simulink model "rtwdemo_codetemplate"  (Simulink 7.6)
settings: Solver=FixedStepDiscrete  StartTime=0.0  StopTime=48  FixedStep=1  RelTol=1e-3
libraries: rtwdemowidgets x2, simulink x1
Description:
  | Formatting Generated Files with Templates
settings Model: Creator=The MathWorks Inc.  ModifiedHistory=This text maps to the Code Template %<ModifiedComment> symbol.  ParamWorkspaceSource=ReferencedWorkspace  CovMetricSettings=d  ExtModeTrigMode=oneshot  ExtModeArmWhenConnect=off  ExtModeAutoUpdateStatusClock=off
settings MATStruct: SampleTime=1  Offset=0  Priority=[20.0]
settings DataIOCC: LimitDataPoints=off  SaveFormat=StructureWithTime  SaveOutput=off  SaveTime=off  SignalLoggingName=sigsOut
settings OptimizationCC: InlineParams=on  InlineInvariantSignals=on  PassReuseOutputArgsAs=Individual arguments  StateBitsets=on  DataBitsets=on  UseTempVars=on  ZeroExternalMemoryAtStartup=off  ZeroInternalMemoryAtStartup=off  NoFixptDivByZeroProtection=on  EfficientFloat2IntCast=on  EfficientMapNaN2IntZero=off  OptimizeModelRefInitCode=on  LifeSpan=1  BufferReusableBoundary=off
settings DebuggingCC: CheckExecutionContextPreStartOutputMsg=on  CheckExecutionContextRuntimeOutputMsg=on  SolverPrmCheckMsg=none  IntegerOverflowMsg=none  StrictBusMsg=ErrorOnBusTreatedAsVector
settings HardwareCC: ProdIntDivRoundTo=Zero  ProdEndianess=LittleEndian  ProdHWDeviceType=Generic->32-bit Embedded Processor  TargetHWDeviceType=Generic->32-bit Embedded Processor
settings ModelReferenceCC: UpdateModelReferenceTargets=IfOutOfDate
settings RTWCC: SystemTargetFile=ert.tlc  TLCOptions=-p0 -aWarnNonSaturatedBlocks=0  TemplateMakefile=ert_default_tmf  Description=Real-Time Workshop Embedded Coder (no auto configuration)  GenerateReport=on  RTWVerbose=off  ProcessScript=ert_make_rtw_hook  IncludeHyperlinkInReport=on  LaunchReport=on
settings CodeAppCC: ForceParamTrailComments=on  IgnoreCustomStorageClasses=off  IgnoreTestpoints=on  SimulinkDataObjDesc=on  CustomSymbolStrGlobalVar=rt$N$M  CustomSymbolStrType=$N$M  CustomSymbolStrFcn=$N$M$F  CustomSymbolStrMacro=$N$M  InsertBlockDesc=on
settings ERTTargetCC: TargetFcnLib=ansi_tfl_tmw.mat  MultiwordLength=2048  GenerateSampleERTMain=on  IncludeMdlTerminateFcn=off  SupportNonFinite=off  SupportComplex=off  InlinedParameterPlacement=NonHierarchical  ERTSrcFileBannerTemplate=rtwdemocodetemplate.cgt  ERTHdrFileBannerTemplate=rtwdemocodetemplate.cgt  ERTDataSrcFileTemplate=rtwdemocodetemplate.cgt  ERTDataHdrFileTemplate=rtwdemocodetemplate.cgt  ERTCustomFileTemplate=example_file_process.tlc  ConvertIfToSwitch=off

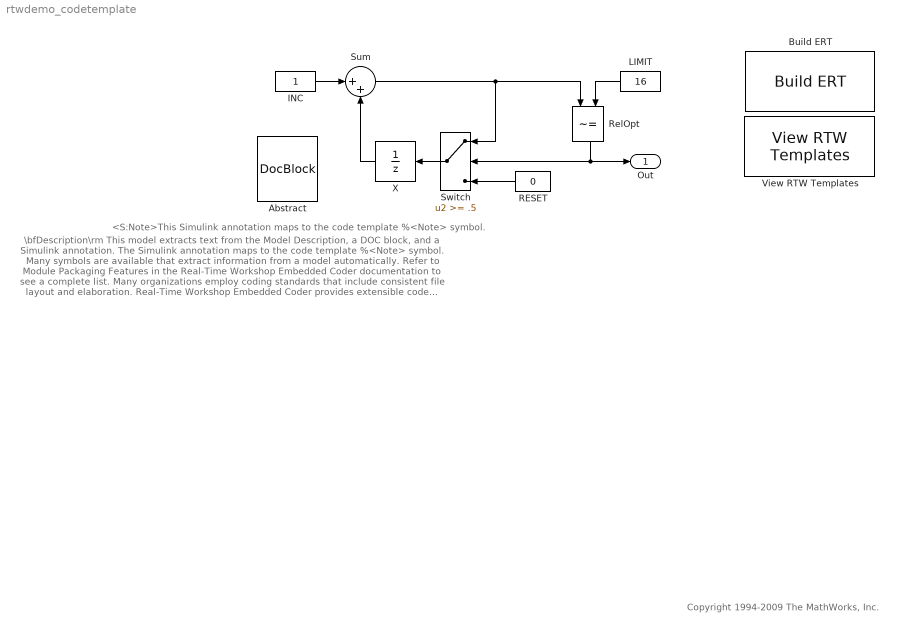
== system rtwdemo_codetemplate ==
  note: \bfDescription\rm
      | This model extracts text from the Model Description, a DOC block, and a Simulink annotation.  The Simulink
      | annotation maps to the code template %<Note> symbol.  Many symbols are available that extract information
      | from a model automatically.  Refer to Module Packaging Features in the Real-Time Workshop Embedded
      | Coder documentation to see a complete list.
      |
      | Many organizations employ coding standards that include consistent file layout and elaboration.  Real-Time
      | Workshop Embedded Coder provides extensible code generation templates for formatting generated code.
      | The layout and format of the code template file controls the output of the generated code.
      |
      | Code generation templates (.cgt files) allow you to add custom code banners, rearrange data and functions,
      | and insert additional code segments and documentation into generated code files.  Code generation
      | templates are picked up automatically from the MATLAB path and employed during the code generation
      | process.  For this model, the code generation template "rtwdemocodetemplate.cgt" is used.
      |
      | \bfInstructions\rm
      | 1. Double-click the yellow View Templates Configuration button to view the templates configuration.
      | 2. Click the Edit button to the right of the "rtwdemocodetemplate.cgt" template, and inspect the code template.
      | 3. Double-click the blue button in the upper right to generate code.  An HTML report appears automatically.
      | 4. Open rtwdemo\_codetemplate.c to inspect the generated code for this model.
  note: <S:Note>This Simulink annotation maps to the code template %<Note> symbol.
  note: Copyright 1994-2009 The MathWorks, Inc.
  Abstract : simulink/Model-Wide Utilities/DocBlock  SystemSampleTime=-1  ECoderFlag=Abstract  DocumentType=Text
      settings: AttributesFormatString=%<ECoderFlag>
  Build ERT : rtwdemowidgets/Build ERT  SystemSampleTime=-1  attrib_overrides={'ERTSrcFileBannerTemplate', 'ERTHdrFileBannerTemplate', 'ERTDataSrcFileTemplate', 'ERTDataHdrFileTemplate'}
  INC : Constant  OutDataTypeStr=uint8
  LIMIT : Constant  Value=16  OutDataTypeStr=uint8
  RESET : Constant  Value=0  OutDataTypeStr=uint8
  RelOpt : RelationalOperator  Operator=~=  InputSameDT=on
  Sum : Sum  Inputs=|++  InputSameDT=on  OutDataTypeStr=Inherit: Same as first input
  Switch : Switch  Threshold=.5  SaturateOnIntegerOverflow=on  InputSameDT=on
  View RTW Templates : rtwdemowidgets/View RTW Templates  SystemSampleTime=-1
  X : UnitDelay  StateIdentifier=X
  Out : Outport
  wires:
  INC/1 -> Sum/1
  X/1 -> Sum/2
  Switch/1 -> X/1
  Sum/1 -> Switch/1, RelOpt/1
  LIMIT/1 -> RelOpt/2
  RESET/1 -> Switch/3
  RelOpt/1 -> Switch/2, Out/1
